simulink model "test"  (R2017b)
settings: Solver=VariableStepAuto  StartTime=0.0  StopTime=10.0  RelTol=1e-3
settings Model: Creator=Student  LastModifiedBy=Student

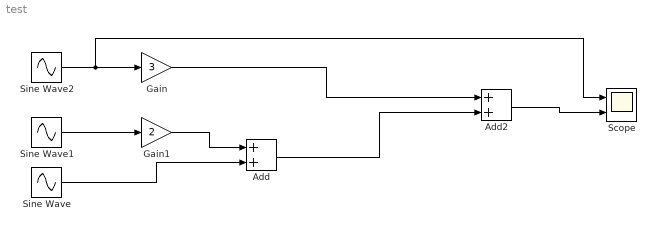
== system test ==
  Add : Sum  Inputs=2
  Add2 : Sum  Inputs=2
  Gain : Gain  Gain=3
  Gain1 : Gain  Gain=2
  Scope : Scope  NumInputPorts=2
  Sine Wave : Sin  SampleTime=0
  Sine Wave1 : Sin  SampleTime=0
  Sine Wave2 : Sin  SampleTime=0
  wires:
  Gain1/1 -> Add/1
  Sine Wave/1 -> Add/2
  Sine Wave1/1 -> Gain1/1
  Sine Wave2/1 -> Scope/1, Gain/1
  Gain/1 -> Add2/1
  Add2/1 -> Scope/2
  Add/1 -> Add2/2
